simulink model "LAB3"  (R2021b)
settings: Solver=VariableStepAuto  StartTime=0.0  StopTime=10.0  RelTol=1e-3
undefined symbols (not defined in the file): J, L
settings Model: Creator=feyzi  LastModifiedBy=feyzi

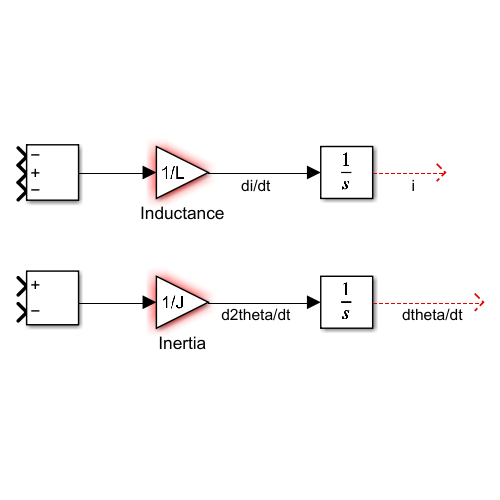
[thumbnail: Simulink's stored preview of the top-level diagram]
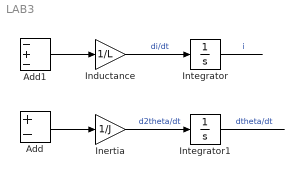
== system LAB3 ==
  Add : Sum  Inputs=+-
  Add1 : Sum  Inputs=-+-
  Inductance : Gain  Gain=1/L
  Inertia : Gain  Gain=1/J
  Integrator : Integrator
  Integrator1 : Integrator
  wires:
  Integrator1/1 -> ?  "dtheta/dt"
  Inertia/1 -> Integrator1/1  "d2theta/dt"
  Integrator/1 -> ?  "i"
  Inductance/1 -> Integrator/1  "di/dt"
  Add/1 -> Inertia/1
  Add1/1 -> Inductance/1
